simulink model "Q3"  (R2020b)
settings: Solver=VariableStepAuto  StartTime=0.0  StopTime=10.0  RelTol=1e-3
libraries: simulink x1
settings Model: Creator=Lenovo  LastModifiedBy=Lenovo

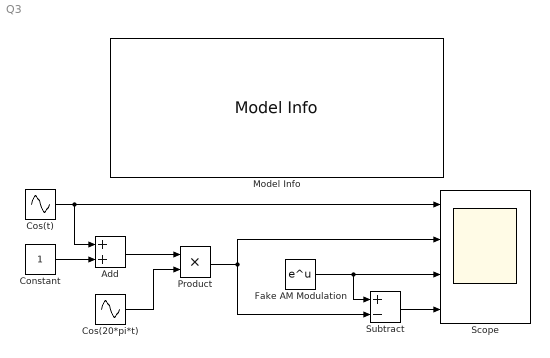
== system Q3 ==
  Add : Sum
  Constant : Constant
  Cos(20*pi*t) : Sin  Frequency=20  Phase=pi/2  SampleTime=0.01
  Cos(t) : Sin  Phase=pi/2  SampleTime=0.01
  Fake AM Modulation : Math  SaturateOnIntegerOverflow=on
  Model Info : simulink/Model-Wide Utilities/Model Info  Frame=on  DisplayStringWithTags=|  HorizontalTextAlignment=Center  LeftAlignmentValue=0.5
      | EE520 Q3 Furkan Sönmez
      | 
      | Cosine wave is derived from sine wave block adding pi/2 phase. 
      | 
      | Cosine Wave Generator
      | Amp = [1 1]
      | Freq= [1 20]
      | Bias = [1 0]
      | Phase =[ pi/2 pi/2]
      | Sample Time =0.01
      | Simulation Duration =10 sec
  Product : Product
  Scope : Scope  NumInputPorts=4
  Subtract : Sum  Inputs=+-
  wires:
  Cos(t)/1 -> Add/1, Scope/1
  Add/1 -> Product/1
  Cos(20*pi*t)/1 -> Product/2
  Constant/1 -> Add/2
  Product/1 -> Scope/2, Subtract/2
  Fake AM Modulation/1 -> Scope/3, Subtract/1
  Subtract/1 -> Scope/4
